simulink model "DEPREMSIGNAL_PID"  (R2024b)
settings: Solver=ode3  StartTime=0.0  StopTime=27.2  FixedStep=0.04  RelTol=1e-3  EnableMultiTasking=on
libraries: arduinolib x6, arduinosensorlib x2
settings Model: ExtModeTrigDuration=2  Creator=cagla  LastModifiedBy=Asus
settings SolverCC: AutoInsertRateTranBlk=on
settings DataIOCC: ReturnWorkspaceOutputs=off
settings OptimizationCC: EnhancedBackFolding=on  PassReuseOutputArgsAs=Individual arguments  ZeroExternalMemoryAtStartup=off  ZeroInternalMemoryAtStartup=off  MaxStackSize=64  OptimizeBlockOrder=speed  DifferentSizesBufferReuse=on  OptimizationCustomize=off  EfficientTunableParamExpr=on
settings DebuggingCC: ParameterTunabilityLossMsg=error
settings HardwareCC: ProdBitPerInt=16  ProdBitPerPointer=16  ProdBitPerSizeT=16  ProdBitPerPtrDiffT=16  ProdLargestAtomicFloat=None  ProdWordSize=8  ProdHWDeviceType=Atmel->AVR
settings SFSimCC: MATLABDynamicMemAlloc=off
settings RTWCC: Description=Embedded Coder  SystemTargetFile=ert.tlc  HardwareBoard=Arduino Mega 2560  TemplateMakefile=ert_default_tmf  Toolchain=Arduino AVR  BuildConfiguration=Faster Runs
settings CodeAppCC: ForceParamTrailComments=on  IgnoreCustomStorageClasses=off  OperatorAnnotations=on  SimulinkDataObjDesc=on  SFDataObjDesc=on  InsertBlockDesc=on
settings ERTTargetCC: SupportContinuousTime=on  SupportNonInlinedSFcns=on  SupportVariableSizeSignals=on  ExtModeTransport=3  ExtModeStaticAlloc=on  ExtModeAutomaticAllocSize=off  ExtModeStaticAllocSize=2048  ExtModeMexFile=ext_xcp  ExtModeIntrfLevel=Level2 - Open  InlinedParameterPlacement=Hierarchical

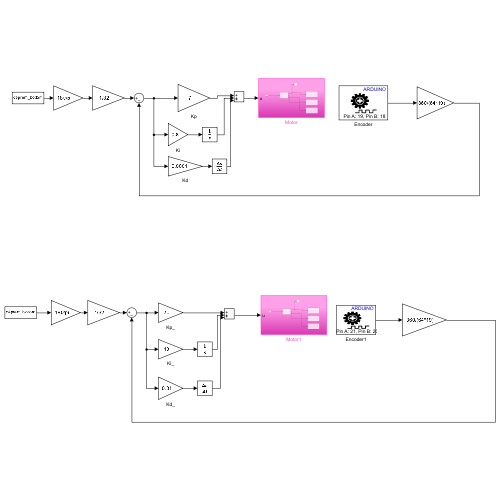
[thumbnail: Simulink's stored preview of the top-level diagram]
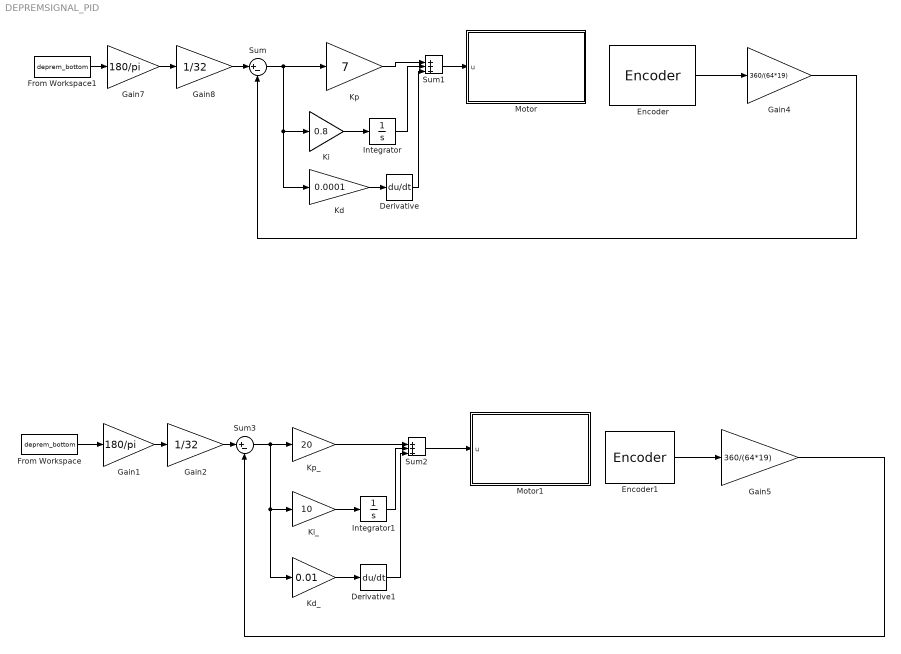
== system DEPREMSIGNAL_PID ==
  Derivative : Derivative
  Derivative1 : Derivative
  Encoder : arduinosensorlib/Encoder  InputA=19  InputB=18  Mode=No reset  SampleTime=-1
      settings: SourceProductName=Sensors
  Encoder1 : arduinosensorlib/Encoder  InputA=21  InputB=20  Mode=No reset  SampleTime=-1
      settings: SourceProductName=Sensors
  From Workspace : FromWorkspace  VariableName=deprem_bottom
  From Workspace1 : FromWorkspace  VariableName=deprem_bottom
  Gain1 : Gain  Gain=180/pi
  Gain2 : Gain  Gain=1/32
  Gain4 : Gain  Gain=360/(64*19)
  Gain5 : Gain  Gain=360/(64*19)
  Gain7 : Gain  Gain=180/pi
  Gain8 : Gain  Gain=1/32
  Integrator : Integrator
  Integrator1 : Integrator
  Kd : Gain  Gain=0.0001
  Kd_ : Gain  Gain=0.01
  Ki : Gain  Gain=0.8
  Ki_ : Gain  Gain=10
  Kp : Gain  Gain=7
  Kp_ : Gain  Gain=20
  Motor : Subsystem
  Motor1 : Subsystem
  Sum : Sum  Inputs=|+-
  Sum1 : Sum  Inputs=|+++
  Sum2 : Sum  Inputs=|+++
  Sum3 : Sum  Inputs=|+-
  wires:
  Sum3/1 -> Kd_/1, Ki_/1, Kp_/1
  Encoder1/1 -> Gain5/1
  Gain4/1 -> Sum/2
  Gain5/1 -> Sum3/2
  Sum/1 -> Kd/1, Ki/1, Kp/1
  Encoder/1 -> Gain4/1
  Gain1/1 -> Gain2/1
  From Workspace/1 -> Gain1/1
  Gain2/1 -> Sum3/1
  Kp_/1 -> Sum2/1
  Sum2/1 -> Motor1/1(u)
  Ki_/1 -> Integrator1/1
  Integrator1/1 -> Sum2/2
  Derivative1/1 -> Sum2/3
  Kd_/1 -> Derivative1/1
  Gain7/1 -> Gain8/1
  From Workspace1/1 -> Gain7/1
  Kp/1 -> Sum1/1
  Sum1/1 -> Motor/1(u)
  Ki/1 -> Integrator/1
  Integrator/1 -> Sum1/2
  Kd/1 -> Derivative/1
  Derivative/1 -> Sum1/3
  Gain8/1 -> Sum/1

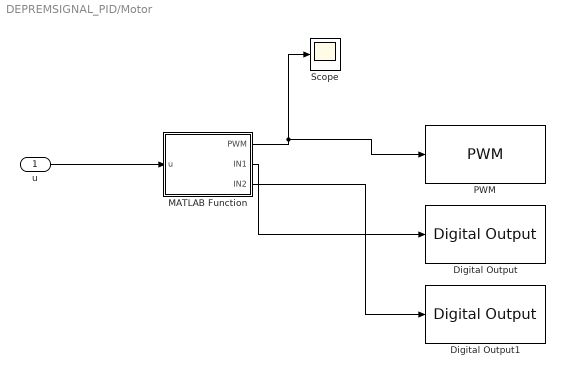
== system DEPREMSIGNAL_PID/Motor ==
  u : Inport
  Digital Output : arduinolib/Digital Output  pinNumber=6  Direction=output  blockPlatform=arduino
      settings: SourceProductName=Common
  Digital Output1 : arduinolib/Digital Output  pinNumber=5  Direction=output  blockPlatform=arduino
      settings: SourceProductName=Common
  MATLAB Function : MATLAB Function  TreatAsAtomicUnit=on
  PWM : arduinolib/PWM  pinNumber=7  frequencyType=Default  desiredFrequency=490.2  achievableFrequency=490.2
      settings: SourceProductName=Common
  Scope : Scope
  wires:
  MATLAB Function/2(IN1) -> Digital Output/1
  MATLAB Function/1(PWM) -> Scope/1, PWM/1
  MATLAB Function/3(IN2) -> Digital Output1/1
  u/1 -> MATLAB Function/1(u)

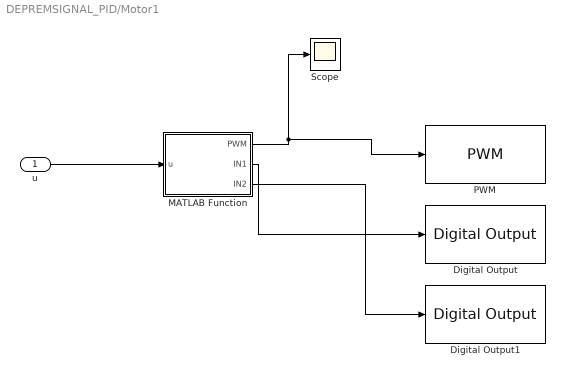
== system DEPREMSIGNAL_PID/Motor1 ==
  u : Inport
  Digital Output : arduinolib/Digital Output  pinNumber=10  Direction=output  blockPlatform=arduino
      settings: SourceProductName=Common
  Digital Output1 : arduinolib/Digital Output  pinNumber=11  Direction=output  blockPlatform=arduino
      settings: SourceProductName=Common
  MATLAB Function : MATLAB Function  TreatAsAtomicUnit=on
  PWM : arduinolib/PWM  pinNumber=9  frequencyType=Default  desiredFrequency=490.2  achievableFrequency=490.2
      settings: SourceProductName=Common
  Scope : Scope
  wires:
  MATLAB Function/2(IN1) -> Digital Output/1
  MATLAB Function/1(PWM) -> Scope/1, PWM/1
  MATLAB Function/3(IN2) -> Digital Output1/1
  u/1 -> MATLAB Function/1(u)

== matlab function DEPREMSIGNAL_PID/Motor1/MATLAB Function ==
  data: u input; PWM output; IN1 output; IN2 output
function [PWM,IN1,IN2] = fcn(u)
PWM=abs(u);
if u<0
    IN1=1;
    IN2=0;
elseif u>0
    IN1=0;
    IN2=1;
else
    IN1=0;
    IN2=0;
end

== matlab function DEPREMSIGNAL_PID/Motor/MATLAB Function ==
  data: u input; PWM output; IN1 output; IN2 output
function [PWM,IN1,IN2] = fcn(u)
PWM=abs(u);
if u<0
    IN1=1;
    IN2=0;
elseif u>0
    IN1=0;
    IN2=1;
else
    IN1=0;
    IN2=0;
end
